simulink model "courseFollow_plant_th"  (R2018b)
settings: Solver=VariableStepAuto  StartTime=0.0  StopTime=end_time  MaxStep=1  RelTol=1e-3
values from neighbouring files (symbols this model uses):
  aB = 1    [courseFollow_plant_ts.m]
  bB = 1    [courseFollow_plant_ts.m]
  initPos = [path7(1);path7(2);path7(3);]    [courseFollow_plant_ts.m]
  phi_curve = .5    (= 0.5)    [courseFollow_plant_ts.m]
libraries: schmehlTangentRotation_ul x1, vectorNormalizer_ul x1, courseFollow_cl x1
settings Model: Creator=jldanie5  LastModifiedBy=jldanie5

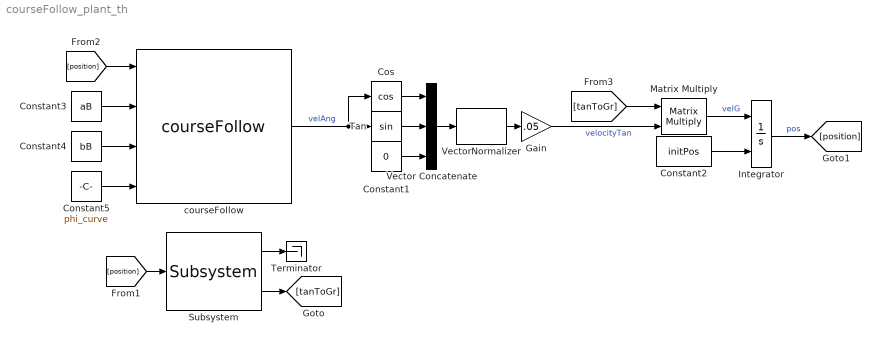
== system courseFollow_plant_th ==
  Constant1 : Constant  Value=0
  Constant2 : Constant  Value=initPos
  Constant3 : Constant  Value=aB
  Constant4 : Constant  Value=bB
  Constant5 : Constant  Value=phi_curve
  Cos : Trigonometry  Operator=cos
  Gain : Gain  Gain=.05
  Integrator : Integrator  InitialConditionSource=external
  Matrix Multiply : Product  Multiplication=Matrix(*)
  Subsystem : schmehlTangentRotation_ul/Subsystem  SystemSampleTime=-1
  Tan : Trigonometry
  Terminator : Terminator
  Vector Concatenate : Concatenate  NumInputs=3
  "VectorNormalizer " : vectorNormalizer_ul/VectorNormalizer   SystemSampleTime=-1
  courseFollow : courseFollow_cl/courseFollow  SystemSampleTime=-1
  wires:
  Subsystem/1 -> Terminator/1
  Subsystem/2 -> [tanToGr]
  Matrix Multiply/1 -> Integrator/1  "velG"
  Constant2/1 -> Integrator/2
  Integrator/1 -> [position]  "pos"
  [position] -> Subsystem/1
  [position] -> courseFollow/1
  Constant3/1 -> courseFollow/2
  Constant4/1 -> courseFollow/3
  Constant5/1 -> courseFollow/4
  [tanToGr] -> Matrix Multiply/1
  Gain/1 -> Matrix Multiply/2  "velocityTan"
  "VectorNormalizer "/1 -> Gain/1
  Constant1/1 -> Vector Concatenate/3
  Cos/1 -> Vector Concatenate/1
  Tan/1 -> Vector Concatenate/2
  courseFollow/1 -> Cos/1, Tan/1  "velAng"
  Vector Concatenate/1 -> "VectorNormalizer "/1
